simulink model "mpc_model_delayed"  (R2019a)
settings: Solver=FixedStepAuto  StartTime=0.0  StopTime=Tfinal  RelTol=1e-3
values from neighbouring files (symbols this model uses):
  A = [-0.0285 -0.0014; -0.0371 -0.1476]    [model.m]
  DCLINK_Cap = 1000e-12    (= 1e-09)    [mpc_model_parameters.m]    (also in mpc_model_parameters_dual_module.m = 0.001)
  FaultTime = 50    [mpc_model_parameters.m]
  FluxPM = MeanInducedVoltagePeak/(2*pi*100)    [mpc_model_parameters.m]    (also in mpc_model_parameters_dual_module.m)
  Inertia = 1e-2    (= 0.01)    [mpc_model_parameters.m]    (also in mpc_model_parameters_dual_module.m)
  Ls = 3.5e-3    (= 0.0035)    [MPC_id_iq.m]    (also in mpc_model_parameters.m = 0.00351; mpc_model_parameters_dual_module.m = 0.00343)
  PolePairs = 10    [mpc_model_parameters.m]    (also in mpc_model_parameters_dual_module.m)
  Rin = 1e-3    (= 0.001)    [mpc_model_parameters.m]    (also in mpc_model_parameters_dual_module.m)
  Rs = 0.531    [Loss_Distribution.m]    (also in MPC_id_iq.m; mpc_model_parameters.m = 0.321; mpc_model_parameters_dual_module.m = 0.539)
  Sampling_time = 1e-6    (= 1e-06)    [mpc_model_parameters.m]    (also in mpc_model_parameters_dual_module.m)
  SpeedRef1 = 50    [mpc_model_parameters.m]    (also in mpc_model_parameters_dual_module.m = 35)
  SpeedRef2 = 100    [mpc_model_parameters.m]    (also in mpc_model_parameters_dual_module.m = 35)
  SpeedRefUpdateTime = 0.25    [mpc_model_parameters.m]    (also in mpc_model_parameters_dual_module.m = 1.75)
  Tload1 = 5    [mpc_model_parameters.m]    (also in mpc_model_parameters_dual_module.m = 30)
  Tload2 = 10    [mpc_model_parameters.m]    (also in mpc_model_parameters_dual_module.m = 63.6619772368)
  TloadUpdateTime = 0.5    [mpc_model_parameters.m]    (also in mpc_model_parameters_dual_module.m)
  Vdc = 50    [mpc_model_parameters.m]    (also in mpc_model_parameters_dual_module.m = 40)
  Vin = Vdc + Rin*(Pout/Vdc)    (= 50.04)    [mpc_model_parameters.m]    (also in mpc_model_parameters_dual_module.m = 40.05)
  ViscousFriction = 1e-3    (= 0.001)    [mpc_model_parameters.m]    (also in mpc_model_parameters_dual_module.m)
undefined symbols (not defined in the file or in its folder): DiscIntNeverNeededParam
libraries: powerlib x16, dspsigops x16, dspswit3 x10, powerlib_meascontrol x3, dspstat3 x3, simulink x2
settings Model: Creator=hakan  LastModifiedBy=hakan
settings SolverCC: ZeroCrossAlgorithm=Adaptive
settings DebuggingCC: IgnoredZcDiagnostic=none

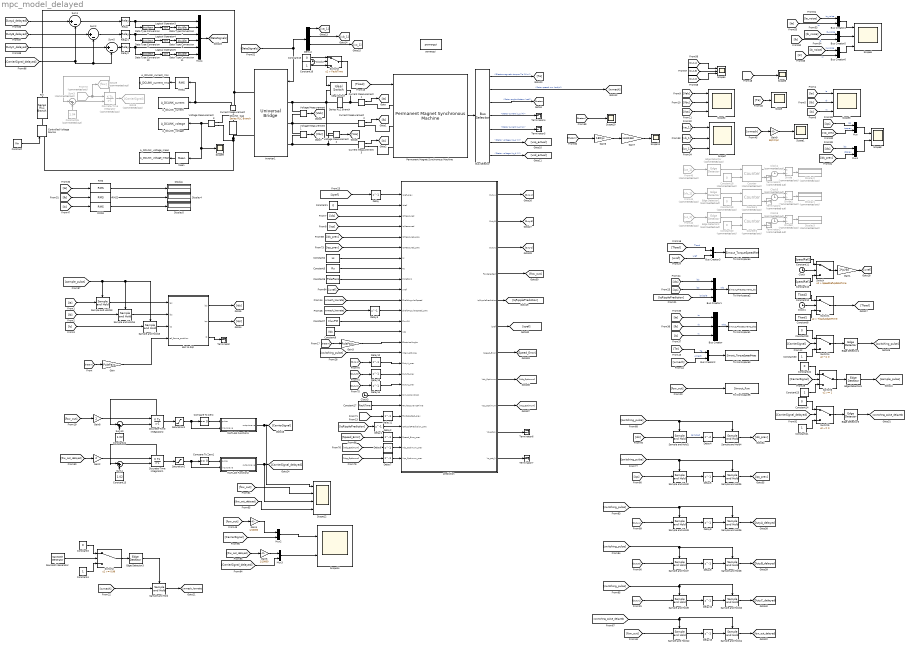
== system mpc_model_delayed ==
  A_DCLINK_current : ToWorkspace  VariableName=A_DCLINK_current  SaveFormat=Structure With Time  SampleTime=-1
  A_DCLINK_current_rms : ToWorkspace  VariableName=A_DCLINK_current_rms  SaveFormat=Structure With Time  SampleTime=-1
  A_DCLINK_voltage : ToWorkspace  VariableName=A_DCLINK_voltage  SaveFormat=Structure With Time  SampleTime=-1
  A_DCLINK_voltage_mean : ToWorkspace  VariableName=A_DCLINK_voltage_mean  SaveFormat=Structure With Time  SampleTime=-1
  Bus Creator : BusCreator  Inputs=3
  Bus Creator1 : BusCreator  Inputs=3
  Bus Creator{2..6} (5 alike) : BusCreator  Inputs=2
  Bus Selector : BusSelector  OutputSignals=Electromagnetic torque Te (N*m),Rotor speed wm (rad/s),Rotor angle thetam (rad),Stator current is_q (A),Stator current is_d (A),Stator voltage Vs_q (V),Stator voltage Vs_d (V)
  Clock{,1..3} (4 alike) : Clock
  Clock4 : Clock  Commented=on
  Clock5 : Clock  Commented=on
  Clock6 : Clock  Commented=on
  Compare To Zero : simulink/Logic and Bit Operations/Compare To Zero  relop===  OutDataTypeStr=boolean
  Compare To Zero1 : simulink/Logic and Bit Operations/Compare To Zero  relop===  OutDataTypeStr=boolean
  Constant : Constant  Value=Vin
  Constant{1,3,14..15,22,29} (6 alike) : Constant  Value=0
  Constant10 : Constant  Value=SpeedRef1
  Constant11 : Constant  Value=SpeedRef2
  Constant12 : Constant  Value=Tload2
  Constant13 : Constant  Value=1.02
  Constant{4,16,21,23,30} (5 alike) : Constant
  Constant17 : Constant  Value=FaultTime
  Constant18 : Constant  Commented=on  Value=0
  Constant19 : Constant  Commented=on  Value=0
  Constant2 : Constant  Value=Ls
  Constant20 : Constant  Commented=on  Value=0
  Constant24 : Constant  Value=1.02
  Constant26 : Constant  Commented=on  Value=1.04
  Constant5 : Constant  Value=Rs
  Constant6 : Constant  Value=PolePairs
  Constant7 : Constant  Value=FluxPM
  Constant8 : Constant  Value=Tload1
  Constant9 : Constant  Value=Vdc
  Controlled Voltage Source : powerlib/Electrical Sources/Controlled Voltage Source  Initialize=on  Source_Type=DC  Amplitude=Vin  Phase=0  Frequency=0  Measurements=None
      settings: SourceProductName=Simscape Electrical
  Counter : dspswit3/Counter  Commented=on  Direction=Up  CountEvent=Rising edge  CounterSize=User defined  MaxCount=9999999999999999999  InitialCount=0  Output=Count and Hit  HitValue=32  ResetInput=on  SamplesPerFrame=1  Ts=1  CntDtype=double  HitDtype=Logical
  Counter1 : dspswit3/Counter  Commented=on  Direction=Up  CountEvent=Rising edge  CounterSize=User defined  MaxCount=9999999999999999999  InitialCount=0  Output=Count and Hit  HitValue=32  ResetInput=on  SamplesPerFrame=1  Ts=1  CntDtype=double  HitDtype=Logical
  Counter2 : dspswit3/Counter  Commented=on  Direction=Up  CountEvent=Rising edge  CounterSize=User defined  MaxCount=9999999999999999999  InitialCount=0  Output=Count and Hit  HitValue=32  ResetInput=on  SamplesPerFrame=1  Ts=1  CntDtype=double  HitDtype=Logical
  Current Measurement{,1..3} (4 alike) : powerlib/Measurements/Current Measurement  PhasorSimulation=off  OutputType=Complex  PSBequivalent=0
      settings: SourceProductName=Simscape Electrical
  DCLINK_Cap : powerlib/Elements/Series RLC Branch  LConnTagsString=__new0  RConnTagsString=__new0  BranchType=C  Resistance=1  Inductance=1e-3  SetiL0=off  InitialCurrent=0  Capacitance=DCLINK_Cap  Setx0=on  InitialVoltage=Vin  Measurements=None
      settings: SourceProductName=Simscape Electrical
  Data Type Conversion10 : DataTypeConversion  OutDataTypeStr=boolean
  Data Type Conversion11 : DataTypeConversion  OutDataTypeStr=double
  Data Type Conversion6 : DataTypeConversion  OutDataTypeStr=boolean
  Data Type Conversion7 : DataTypeConversion  OutDataTypeStr=double
  Data Type Conversion8 : DataTypeConversion  OutDataTypeStr=boolean
  Data Type Conversion9 : DataTypeConversion  OutDataTypeStr=double
  Delay{,1..3,5..15} (15 alike) : Delay  DelayLength=1
  Delay4 : Delay
  Demux : Demux  Outputs=6
  Discrete-Time Integrator : DiscreteIntegrator  Commented=on  ExternalReset=falling  SampleTime=-1  ShowStatePort=on  ICPrevOutput=DiscIntNeverNeededParam  ICPrevScaledInput=DiscIntNeverNeededParam
  Discrete-Time Integrator1 : DiscreteIntegrator  ExternalReset=falling  SampleTime=Sampling_time  UpperSaturationLimit=1  LowerSaturationLimit=0  ShowStatePort=on  ICPrevOutput=DiscIntNeverNeededParam  ICPrevScaledInput=DiscIntNeverNeededParam
  Discrete-Time Integrator2 : DiscreteIntegrator  ExternalReset=falling  SampleTime=Sampling_time  UpperSaturationLimit=1  LowerSaturationLimit=0  ShowStatePort=on  ICPrevOutput=DiscIntNeverNeededParam  ICPrevScaledInput=DiscIntNeverNeededParam
  Display : Display
  Display1 : Display  Commented=on
  Display2 : Display  Commented=on
  Display3 : Display  Commented=on
  Display4 : Display
  Display5 : Display
  Divide : Product  Commented=on  Inputs=*/
  Divide1 : Product  Commented=on  Inputs=*/
  Divide2 : Product  Commented=on  Inputs=*/
  Edge Detector : dspswit3/Edge Detector  Commented=on  InputProcessing=Columns as channels (frame based)
      settings: SourceProductName=DSP System Toolbox  SourceProductBaseCode=DS
  Edge Detector1 : dspswit3/Edge Detector  Commented=on  InputProcessing=Columns as channels (frame based)
      settings: SourceProductName=DSP System Toolbox  SourceProductBaseCode=DS
  Edge Detector2 : dspswit3/Edge Detector  Commented=on  InputProcessing=Columns as channels (frame based)
      settings: SourceProductName=DSP System Toolbox  SourceProductBaseCode=DS
  Edge Detector{3..6} (4 alike) : dspswit3/Edge Detector  InputProcessing=Columns as channels (frame based)
      settings: SourceProductName=DSP System Toolbox  SourceProductBaseCode=DS
  From40 : From  Commented=on  GotoTag=va_1
  From41 : From  Commented=on  GotoTag=vb_1
  From42 : From  Commented=on  GotoTag=vc_1
  From72 : From  Commented=on  GotoTag=fsw_out
  Gain : Gain  Gain=PolePairs
  Gain1 : Gain  Gain=2*pi/60
  Gain2 : Gain  Gain=2
  Gain3 : Gain  Gain=PolePairs
  Gain4 : Gain  Gain=1/10000
  Gain5 : Gain  Gain=1/10000
  Gain6 : Gain  Gain=180/pi
  Gain7 : Gain  Gain=14400/360
  Gain8 : Gain  Gain=2
  Gain9 : Gain  Gain=60/(2*pi)
  Goto29 : Goto  Commented=on  GotoTag=fsw
  Goto9 : Goto  Commented=on  GotoTag=CarrierSignal
  Ideal Switch : powerlib/Power Electronics/Ideal Switch  Ron=0.001  Lon=0  IC=0  Rs=1e5  Cs=inf  Measurements=on
      settings: SourceProductName=Simscape Electrical
  Inverter1 : powerlib/Power Electronics/Universal Bridge  Arms=3  SnubberResistance=1e5  SnubberCapacitance=inf  Device=IGBT / Diodes  Ron=0.65e-3  Lon=0  ForwardVoltages="[  0  0  ]"  ForwardVoltage=0  GTOparameters=[ 10e-6 , 20e-6 ]  IGBTparameters=[ 1e-6 , 2e-6 ]  Measurements=All voltages and currents  Measurements_2=None  converterType=Rectifier
      settings: SourceProductName=Simscape Electrical
  Logical Operator3 : Logic  Operator=NOT  AllPortsSameDT=off  OutDataTypeStr=boolean
  Logical Operator4 : Logic  Operator=NOT  AllPortsSameDT=off  OutDataTypeStr=boolean
  Logical Operator5 : Logic  Operator=NOT  AllPortsSameDT=off  OutDataTypeStr=boolean
  MATLAB Function1 : MATLAB Function  TreatAsAtomicUnit=on
  MATLAB Function2 : MATLAB Function  TreatAsAtomicUnit=on
  Mean : powerlib_meascontrol/Measurements/Mean  Freq=THD_mean_frequency  Vinit=0  Ts=0
      settings: SourceProductName=Simscape Electrical
  Mux{,1..3} (4 alike) : Mux  Inputs=2
  Mux4 : Mux  Inputs=6
  Permanent Magnet Synchronous Machine : powerlib/Machines/Permanent Magnet Synchronous Machine  NbPhases=3  FluxDistribution=Sinusoidal  RotorType=Round  MechanicalLoad=Torque Tm  PresetModel=No  ShowDetailedParameters=on  MeasurementBus=off  Resistance=Rs  Inductance=8.5e-3  dqInductances=[3.1e-3,3.6e-3]  La=Ls_Machine  MachineConstant=Voltage Constant (V_peak L-L / krpm)  Flux=0.18074  VoltageCst=VoltageConstant  TorqueCst=2.7111  Flat=120  Mechanical=[Inertia ViscousFriction PolePairs 0]  PolePairs=4  InitialConditions=[0*100*2*pi/60,0, 0,0]  InitialConditions5ph=[0 0 0 0 0 0]  TsPowergui=0  TsBlock=-1  RefAngle=90 degrees behind phase A axis (modified Park)
  RMS : dspstat3/RMS  run=off  directionMode=Each column  dimension=1  InputProcessing=Columns as channels (frame based)  reset_popup=None
  RMS1 : powerlib_meascontrol/Measurements/RMS  TrueRMS=on  Freq=Load_Nominal_Freq  RMSInit=10  Ts=0
      settings: SourceProductName=Simscape Electrical
  RMS2 : dspstat3/RMS  run=off  directionMode=Each column  dimension=1  InputProcessing=Columns as channels (frame based)  reset_popup=None
  RMS3 : dspstat3/RMS  run=off  directionMode=Each column  dimension=1  InputProcessing=Columns as channels (frame based)  reset_popup=None
  Relay : Relay
  Relay1 : Relay
  Relay2 : Relay
  Rin : powerlib/Elements/Series RLC Branch  LConnTagsString=__new0  RConnTagsString=__new0  BranchType=R  Resistance=Rin  Inductance=1e-3  SetiL0=off  InitialCurrent=0  Capacitance=1000e-6  Setx0=off  InitialVoltage=0  Measurements=None
      settings: SourceProductName=Simscape Electrical
  Sample and Hold{,1..15} (16 alike) : dspsigops/Sample and Hold  trig=Rising edge  initCond=0  latchinput=off
  Saturation1 : Saturate  UpperLimit=1  LowerLimit=0
  Saturation2 : Saturate  UpperLimit=1  LowerLimit=0
  Sawtooth Generator : powerlib_meascontrol/Pulse & Signal Generators/Sawtooth Generator  Freq=100  Phase=180  Ts=0
      settings: SourceProductName=Simscape Electrical
  Scope{,1,5,9..11} (6 alike) : Scope
  Scope12 : Scope  NumInputPorts=4
  Scope14 : Scope  NumInputPorts=2
  Scope{2..4,6..7} (5 alike) : Scope  NumInputPorts=3
  Scope8 : Scope  NumInputPorts=2
  Series RLC Branch : powerlib/Elements/Series RLC Branch  LConnTagsString=__new0  RConnTagsString=__new0  BranchType=R  Resistance=5000  Inductance=1e-3  SetiL0=off  InitialCurrent=0  Capacitance=1e-6  Setx0=off  InitialVoltage=0  Measurements=None
      settings: SourceProductName=Simscape Electrical
  Sum1 : Sum  Inputs=|+-
  Sum10 : Sum  Inputs=|-+
  Sum2 : Sum  Inputs=|+-
  Sum3 : Sum  Commented=on  Inputs=|-+
  Sum4 : Sum  Inputs=|-+
  Sum5 : Sum  Inputs=|+-
  Switch : Switch  Criteria=u2 > Threshold  Threshold=SpeedRefUpdateTime
  Switch1 : Switch  Criteria=u2 > Threshold  Threshold=TloadUpdateTime
  Switch2 : Switch  Threshold=0.99
  Switch3 : Switch  Criteria=u2 > Threshold  Threshold=FaultTime
  Switch4 : Switch  Criteria=u2 ~= 0
  Switch5 : Switch  Criteria=u2 ~= 0
  Switch6 : Switch  Threshold=1
  Terminator{,4..7} (5 alike) : Terminator
  Terminator1 : Terminator  Commented=on
  Terminator2 : Terminator  Commented=on
  Terminator3 : Terminator  Commented=on
  To Workspace1 : ToWorkspace  VariableName=Simout_PhaseCurrents_abc  SaveFormat=Timeseries  SampleTime=-1
  To Workspace2 : ToWorkspace  VariableName=Simout_PhaseCurrents_dq  SaveFormat=Timeseries  SampleTime=-1
  To Workspace3 : ToWorkspace  VariableName=Simout_TorqueSpeedMeas  SaveFormat=Timeseries  SampleTime=-1
  To Workspace4 : ToWorkspace  VariableName=Simout_TorqueSpeedRef  SaveFormat=Timeseries  SampleTime=-1
  To Workspace5 : ToWorkspace  VariableName=Simout_Fsw  SaveFormat=Timeseries  SampleTime=-1
  Voltage Measurement{,1..3} (4 alike) : powerlib/Measurements/Voltage Measurement  PhasorSimulation=off  OutputType=Complex  PSBequivalent=0
      settings: SourceProductName=Simscape Electrical
  abc to dq0 : MATLAB Function  TreatAsAtomicUnit=on
  powergui : powerlib/powergui  Priority=1  SimulationMode=Discrete  SampleTime=Sampling_time  frequency=60  Iterations=50  frequencyindice=0  Pbase=100e6  ErrMax=1e-4  UnitsV=kV  UnitsW=MW  buscounter=0  FunctionMessages=off  echomessages=off  EnableUseOfTLC=off  CurrentSourceSwitches=off  DisableSnubberDevices=off  DisableRonSwitches=off  DisableVfSwitches=off  DisplayEquations=off  AutomaticDiscreteSolvers=off  SolverType=Tustin/Backward Euler (TBE)  Interpol=off  ExternalGateDelay=off  methode=off  Ts=100  x0status=blocks  SPID=on  SwTol=0  HookPort=off  NonlinearTolerance=0  nMaxIteration=15  ContinueOnMaxIteration=off  RestoreLinks=warning  ResistiveCurrentMeasurement=off  Frange=[0:2:500]  Ylog=off  Xlog=on  ShowGrid=off  save=off  variable=ZData  structure=0  ZoomFFT=off  StartTime=0.0  cycles=1  DisplayStyle=1  fundamental=60  FreqAxis=off  MaxFrequency=1000  frequencyindicesteady=1  RmsSteady=1  display=off
      settings: SourceProductName=Simscape Electrical
  prediction : MATLAB Function  TreatAsAtomicUnit=on
  wires:
  Voltage Measurement3/1 -> Scope9/1, Mean/1, A_DCLINK_voltage/1
  RMS1/1 -> A_DCLINK_current_rms/1
  Constant/1 -> Controlled Voltage Source/1
  Mean/1 -> A_DCLINK_voltage_mean/1
  Current Measurement/1 -> RMS1/1, A_DCLINK_current/1
  Permanent Magnet Synchronous Machine/1 -> Bus Selector/1
  Bus Selector/1 -> [Te]  "<Electromagnetic torque Te (N*m)>"
  Bus Selector/2 -> [wmech]  "<Rotor speed wm (rad/s)>"
  Current Measurement1/1 -> [Ia]
  Current Measurement2/1 -> [Ib]
  Current Measurement3/1 -> [Ic]
  Bus Selector/3 -> [thetam]  "<Rotor angle thetam (rad)>"
  Bus Selector/4 -> Terminator4/1  "<Stator current is_q (A)>"
  Bus Selector/5 -> Terminator5/1  "<Stator current is_d (A)>"
  [ids] -> prediction/3(IdMeasured)
  [iqs] -> prediction/4(IqMeasured)
  Constant2/1 -> prediction/7(Ls)
  Voltage Measurement/1 -> [Vab]
  Voltage Measurement1/1 -> [Vbc]
  Voltage Measurement2/1 -> [Vca]
  Bus Selector/6 -> [vsq_actual]  "<Stator voltage Vs_q (V)>"
  Bus Selector/7 -> [vsd_actual]  "<Stator voltage Vs_d (V)>"
  [Vca] -> Scope2/3
  [Vbc] -> Scope2/2
  [Vab] -> Scope2/1
  Constant5/1 -> prediction/8(Rs)
  Constant6/1 -> prediction/9(PolePairs)
  [wmech_lowrate] -> prediction/11(ShaftAngularSpeed)
  Constant7/1 -> prediction/13(FluxPM)
  Constant9/1 -> prediction/14(Vdc)
  Gain3/1 -> prediction/15(ElectricalAngle)
  [thetam] -> Gain3/1
  [Tload] -> Permanent Magnet Synchronous Machine/1
  [iqs] -> Bus Creator1/2  "iqs"
  [ids] -> Bus Creator1/1  "ids"
  Constant10/1 -> Switch/3
  Constant11/1 -> Switch/1
  Switch/1 -> Gain1/1
  Clock/1 -> Switch/2
  Clock1/1 -> Switch1/2
  Constant12/1 -> Switch1/1
  Constant8/1 -> Switch1/3
  Switch1/1 -> [Tload]
  Bus Creator/1 -> To Workspace1/1  "Iabc"
  Bus Creator1/1 -> To Workspace2/1  "Idq"
  Bus Creator2/1 -> To Workspace3/1
  Gain1/1 -> [wref]
  [Tload] -> Bus Creator3/1  "Tload"
  [wref] -> Bus Creator3/2  "wref"
  Bus Creator3/1 -> To Workspace4/1
  [switching_pulse] -> prediction/16(InterruptPulse)
  Clock2/1 -> Switch3/2
  Constant15/1 -> Switch3/1
  Constant16/1 -> Switch3/3
  Switch3/1 -> Ideal Switch/1
  Clock3/1 -> prediction/20(SimulationClock)
  Constant17/1 -> prediction/21(FaultOccuranceTime)
  [va_1] -> Scope7/1
  [vb_1] -> Scope7/2
  [vc_1] -> Scope7/3
  Edge Detector/1 -> Counter/1
  Constant18/1 -> Counter/2
  Counter/1 -> Divide/1
  Clock4/1 -> Divide/2
  Divide/1 -> Display2/1
  [Ib] -> Bus Creator/2  "Ib"
  [Ia] -> Bus Creator/1  "Ia"
  [Ic] -> Bus Creator/3  "Ic"
  [Ib] -> Scope3/2  "Ib"
  [Ic] -> Scope3/3  "Ic"
  [Ia] -> Scope3/1  "Ia"
  Counter/2 -> Terminator1/1
  From40/1 -> Edge Detector/1
  From41/1 -> Edge Detector1/1
  Counter1/2 -> Terminator2/1
  Divide1/1 -> Display1/1
  Clock5/1 -> Divide1/2
  Counter1/1 -> Divide1/1
  Constant19/1 -> Counter1/2
  Edge Detector1/1 -> Counter1/1
  Edge Detector2/1 -> Counter2/1
  Constant20/1 -> Counter2/2
  Counter2/1 -> Divide2/1
  Clock6/1 -> Divide2/2
  Divide2/1 -> Display3/1
  Counter2/2 -> Terminator3/1
  From42/1 -> Edge Detector2/1
  [Te] -> Bus Creator2/1  "Te"
  [wmech] -> Bus Creator2/2  "wmech"
  [Te] -> Scope/1
  [wmech] -> Gain9/1
  prediction/1(DutyA) -> [DutyA]
  prediction/3(DutyC) -> [DutyC]
  prediction/2(DutyB) -> [DutyB]
  [DutyB] -> Scope4/2
  [DutyA] -> Scope4/1
  [DutyC] -> Scope4/3
  Constant26/1 -> Sum3/2
  From72/1 -> Goto29/1, Discrete-Time Integrator/1
  Discrete-Time Integrator/State -> Sum3/1
  Sum3/1 -> Discrete-Time Integrator/2
  Switch4/1 -> Edge Detector4/1
  Constant30/1 -> Switch4/3
  Constant29/1 -> Switch4/1
  [GateSignals] -> Inverter1/1, Demux/1
  Demux/1 -> [va_1]
  Demux/3 -> [vb_1]
  prediction/4(FswSelected) -> [fsw_out]
  Delay11/1 -> prediction/22(FswSelected_prev)
  [fsw_out] -> Delay11/1
  [DutyB] -> Delay13/1
  [DutyA] -> Delay12/1
  [DutyC] -> Delay14/1
  Delay13/1 -> prediction/18(DutyB_prev)
  Delay12/1 -> prediction/17(DutyA_prev)
  Delay14/1 -> prediction/19(DutyC_prev)
  Discrete-Time Integrator/1 -> Goto9/1
  [CarrierSignal] -> Switch4/2
  Demux/5 -> [vc_1]
  [IqRipplePrediction] -> Delay1/1
  Delay1/1 -> prediction/23(IqRipplePrediction_prev)
  [CarrierSignal_delayed] -> Sum2/2, Sum5/2, Sum1/2
  Logical Operator4/1 -> Data Type Conversion9/1
  [DutyA_delayed] -> Sum1/1
  Data Type Conversion8/1 -> Logical Operator4/1
  Data Type Conversion10/1 -> Logical Operator5/1
  Relay1/1 -> Data Type Conversion8/1, Mux4/3
  Relay2/1 -> Data Type Conversion10/1, Mux4/5
  Data Type Conversion6/1 -> Logical Operator3/1
  Sum1/1 -> Relay/1
  Data Type Conversion11/1 -> Mux4/6
  [DutyC_delayed] -> Sum5/1
  Relay/1 -> Mux4/1, Data Type Conversion6/1
  Data Type Conversion9/1 -> Mux4/4
  Sum5/1 -> Relay2/1
  Logical Operator3/1 -> Data Type Conversion7/1
  Logical Operator5/1 -> Data Type Conversion11/1
  Sum2/1 -> Relay1/1
  Mux4/1 -> [GateSignals]
  [DutyB_delayed] -> Sum2/1
  Data Type Conversion7/1 -> Mux4/2
  [fsw_out] -> Scope5/1
  Discrete-Time Integrator2/State -> Sum10/1
  Gain8/1 -> Discrete-Time Integrator2/1
  Sum10/1 -> Discrete-Time Integrator2/2
  [fsw_out] -> Gain8/1
  Saturation1/1 -> MATLAB Function1/2(inputwave), Compare To Zero/1
  Constant24/1 -> Sum10/2
  Discrete-Time Integrator2/1 -> Saturation1/1
  Compare To Zero/1 -> MATLAB Function1/1(pulse)
  MATLAB Function1/1(outputwave) -> Scope12/1, [CarrierSignal]
  [fsw_out] -> To Workspace5/1
  [IqRipplePrediction] -> Bus Creator1/3  "iqripple"
  Constant1/1 -> prediction/2(idref)
  prediction/5(IqRipplePrediction) -> [IqRipplePrediction]
  Switch2/1 -> Edge Detector3/1
  Edge Detector3/1 -> Sample and Hold/Trigger
  Constant4/1 -> Switch2/3
  Sawtooth Generator/1 -> Switch2/2
  Constant3/1 -> Switch2/1
  [wmech] -> Sample and Hold/1
  Sample and Hold/1 -> [wmech_lowrate]
  [Ia] -> RMS/1
  [Ib] -> RMS2/1
  [Ic] -> RMS3/1
  RMS/1 -> Display/1
  RMS2/1 -> Display4/1
  RMS3/1 -> Display5/1
  abc to dq0/2(iqs) -> [iqs]
  Gain/1 -> abc to dq0/4(ref_frame_position)
  abc to dq0/1(ids) -> [ids]
  abc to dq0/3(i0) -> Terminator/1
  [thetam] -> Gain/1
  [Ia_noise] -> Bus Creator4/1  "Ia_noise"
  [Ia] -> Bus Creator4/2  "Ia"
  [Ib] -> Bus Creator5/2  "Ib"
  [Ib_noise] -> Bus Creator5/1  "Ib_noise"
  [Ic_noise] -> Bus Creator6/1  "Ic_noise"
  [Ic] -> Bus Creator6/2  "Ic"
  Bus Creator5/1 -> Scope6/2
  Bus Creator4/1 -> Scope6/1
  Bus Creator6/1 -> Scope6/3
  prediction/6(iqref) -> [iqref]
  Delay/1 -> prediction/1(iqref_prev)
  [iqref] -> Delay/1
  [wref] -> prediction/10(wref)
  [wmech_lowrate] -> Delay3/1
  prediction/7(Speed_Error) -> [Speed_Error]
  Delay2/1 -> prediction/24(Speed_Error_prev)
  [Speed_Error] -> Delay2/1
  Delay3/1 -> prediction/12(ShaftAngularSpeed_prev)
  [thetam] -> Scope10/1
  [thetam] -> Gain6/1
  Gain6/1 -> Gain7/1
  Gain7/1 -> Scope11/1
  Edge Detector4/1 -> [switching_pulse]
  [switching_pulse] -> Sample and Hold4/Trigger, Sample and Hold1/Trigger
  [ids] -> Sample and Hold1/1
  [iqs] -> Sample and Hold2/1
  [switching_pulse] -> Sample and Hold5/Trigger, Sample and Hold2/Trigger
  Sample and Hold1/1 -> Delay4/1  "sampled"
  Sample and Hold2/1 -> Delay5/1
  Delay5/1 -> Sample and Hold5/1
  Delay4/1 -> Sample and Hold4/1
  Sample and Hold4/1 -> [ids_prev]
  Sample and Hold5/1 -> [iqs_prev]
  [ids_prev] -> prediction/5(IdMeasured_prev)
  [iqs_prev] -> prediction/6(IqMeasured_prev)
  prediction/8(Vds_Optimum) -> [Vds_Optimum]
  prediction/9(Vqs_Optimum) -> [Vqs_Optimum]
  [Vds_Optimum] -> Delay6/1
  [Vqs_Optimum] -> Delay7/1
  Delay6/1 -> prediction/25(Vds_Optimum_prev)
  Delay7/1 -> prediction/26(Vqs_Optimum_prev)
  prediction/10(Vd_est_1) -> Terminator6/1
  prediction/11(Vq_est_1) -> Terminator7/1
  Gain9/1 -> Scope1/1
  [iqs] -> Mux/1  "iqs"
  [iqs_prev] -> Mux/2  "iqsprev"
  Mux/1 -> Scope8/1
  Mux1/1 -> Scope8/2
  [ids] -> Mux1/1  "ids"
  [ids_prev] -> Mux1/2  "idsprev"
  Sample and Hold6/1 -> [DutyA_delayed]
  Delay8/1 -> Sample and Hold6/1
  Sample and Hold3/1 -> Delay8/1
  [switching_pulse] -> Sample and Hold6/Trigger, Sample and Hold3/Trigger
  [DutyA] -> Sample and Hold3/1
  [DutyB] -> Sample and Hold7/1
  [switching_pulse] -> Sample and Hold7/Trigger, Sample and Hold8/Trigger
  Sample and Hold7/1 -> Delay9/1
  Delay9/1 -> Sample and Hold8/1
  Sample and Hold8/1 -> [DutyB_delayed]
  Sample and Hold10/1 -> [DutyC_delayed]
  Delay10/1 -> Sample and Hold10/1
  Sample and Hold9/1 -> Delay10/1
  [switching_pulse] -> Sample and Hold10/Trigger, Sample and Hold9/Trigger
  [DutyC] -> Sample and Hold9/1
  [fsw_out] -> Sample and Hold12/1
  [switching_pulse_delayed] -> Sample and Hold11/Trigger, Sample and Hold12/Trigger
  Sample and Hold11/1 -> [fsw_out_delayed]
  Sample and Hold12/1 -> Delay15/1
  Delay15/1 -> Sample and Hold11/1
  MATLAB Function2/1(outputwave) -> Scope12/3, [CarrierSignal_delayed]
  Compare To Zero1/1 -> MATLAB Function2/1(pulse)
  Discrete-Time Integrator1/1 -> Saturation2/1
  Constant13/1 -> Sum4/2
  Saturation2/1 -> Compare To Zero1/1, MATLAB Function2/2(inputwave)
  [fsw_out_delayed] -> Gain2/1
  Sum4/1 -> Discrete-Time Integrator1/2
  Gain2/1 -> Discrete-Time Integrator1/1
  Discrete-Time Integrator1/State -> Sum4/1
  [fsw_out] -> Scope12/2
  [fsw_out_delayed] -> Scope12/4
  Edge Detector5/1 -> [switching_pulse_delayed]
  [CarrierSignal_delayed] -> Switch5/2
  Constant14/1 -> Switch5/1
  Constant21/1 -> Switch5/3
  Switch5/1 -> Edge Detector5/1
  Mux2/1 -> Scope14/1
  Mux3/1 -> Scope14/2
  [fsw_out_delayed] -> Gain5/1
  [fsw_out] -> Gain4/1
  [CarrierSignal] -> Mux2/2
  [CarrierSignal_delayed] -> Mux3/2
  Gain4/1 -> Mux2/1
  Gain5/1 -> Mux3/1
  Edge Detector6/1 -> [sample_pulse]
  [CarrierSignal] -> Switch6/2
  Constant22/1 -> Switch6/1
  Constant23/1 -> Switch6/3
  Switch6/1 -> Edge Detector6/1
  [Ia] -> Sample and Hold13/1
  Sample and Hold13/1 -> abc to dq0/1(ias)
  Sample and Hold14/1 -> abc to dq0/2(ibs)
  [Ib] -> Sample and Hold14/1
  Sample and Hold15/1 -> abc to dq0/3(ics)
  [Ic] -> Sample and Hold15/1
  [sample_pulse] -> Sample and Hold15/Trigger, Sample and Hold14/Trigger, Sample and Hold13/Trigger
  connections:
  Rin/LConn1 -- Current Measurement/RConn1 -- Inverter1/RConn1
  Controlled Voltage Source/LConn1 -- Voltage Measurement3/LConn2 -- DCLINK_Cap/RConn1 -- Inverter1/RConn2
  DCLINK_Cap/LConn1 -- Current Measurement/LConn1 -- Voltage Measurement3/LConn1
  Controlled Voltage Source/RConn1 -- Rin/RConn1
  Voltage Measurement2/LConn2 -- Ideal Switch/LConn1 -- Series RLC Branch/LConn1 -- Voltage Measurement/LConn1 -- Inverter1/LConn1
  Current Measurement2/LConn1 -- Voltage Measurement1/LConn1 -- Voltage Measurement/LConn2 -- Inverter1/LConn2
  Inverter1/LConn3 -- Voltage Measurement1/LConn2 -- Voltage Measurement2/LConn1 -- Current Measurement3/LConn1
  Current Measurement3/RConn1 -- Permanent Magnet Synchronous Machine/LConn3
  Permanent Magnet Synchronous Machine/LConn2 -- Current Measurement2/RConn1
  Permanent Magnet Synchronous Machine/LConn1 -- Current Measurement1/RConn1
  Current Measurement1/LConn1 -- Ideal Switch/RConn1 -- Series RLC Branch/RConn1

== matlab function mpc_model_delayed/prediction ==
  data: DutyA output; DutyB output; DutyC output; iqref_prev input; idref input; IdMeasured input; IqMeasured input; IdMeasured_prev input; IqMeasured_prev input; Ls input; Rs input; PolePairs input; wref input; ShaftAngularSpeed input; ShaftAngularSpeed_prev input; FluxPM input; Vdc input; ElectricalAngle input; InterruptPulse input; DutyA_prev input; DutyB_prev input; DutyC_prev input; SimulationClock input; FaultOccuranceTime input; FswSelected_prev input; FswSelected output; IqRipplePrediction output; IqRipplePrediction_prev input; iqref output; Speed_Error_prev input; Speed_Error output; Vds_Optimum output; Vqs_Optimum output; Vds_Optimum_prev input; Vqs_Optimum_prev input; Vd_est_1 output; Vq_est_1 output
function [DutyA, DutyB, DutyC, FswSelected, IqRipplePrediction,iqref,Speed_Error,Vds_Optimum,Vqs_Optimum,Vd_est_1,Vq_est_1] = fcn(iqref_prev,idref,IdMeasured, IqMeasured, IdMeasured_prev, IqMeasured_prev, Ls, Rs,PolePairs,wref, ShaftAngularSpeed,ShaftAngularSpeed_prev, FluxPM,Vdc,ElectricalAngle,InterruptPulse,DutyA_prev, DutyB_prev, DutyC_prev, SimulationClock,FaultOccuranceTime,FswSelected_prev, IqRipplePrediction_prev,Speed_Error_prev,Vds_Optimum_prev,Vqs_Optimum_prev)
Ld = Ls;
Lq = Ls;
Iq_Rated = 11.7362; %this is the rated value of the IqMeasured
% cost = zeros(1,8);
% VdPrediction_1 = zeros(1,8);
% VqPrediction_1 = zeros(1,8);
% FswOptions = [5000; 10000; 15000; 20000; 25000; 30000; 35000; 40000];
FswMax = 10000;
FswOptions = 1000:1000:FswMax;
cost = zeros(1,numel(FswOptions));
% VdPrediction_1 = zeros(1,numel(FswOptions));
% VqPrediction_1 = zeros(1,numel(FswOptions));
Vd_est_1 = zeros(1,numel(FswOptions));
Vq_est_1 = zeros(1,numel(FswOptions));
% Vd_est_2 = zeros(1,numel(FswOptions));
% Vq_est_2 = zeros(1,numel(FswOptions));
VdPrediction_2 = zeros(1,numel(FswOptions));
VqPrediction_2 = zeros(1,numel(FswOptions));
IqRipplePredictionArray_1 = zeros(1,numel(FswOptions));
IqRipplePredictionArray_2 = zeros(1,numel(FswOptions));
VoltageDuring_T1_1 = zeros(1,numel(FswOptions));
VoltageDuring_T2_1 = zeros(1,numel(FswOptions));
VoltageDuring_T0_1 = zeros(1,numel(FswOptions));
VoltageDuring_T1_2 = zeros(1,numel(FswOptions));
VoltageDuring_T2_2 = zeros(1,numel(FswOptions));
VoltageDuring_T0_2 = zeros(1,numel(FswOptions));
MagnitudePrediction_1 = zeros(1,numel(FswOptions));
MagnitudePrediction_2 = zeros(1,numel(FswOptions));

SvpwmT1Prediction_1 =  zeros(1,numel(FswOptions));
SvpwmT2Prediction_1 =  zeros(1,numel(FswOptions));
SvpwmT0Prediction_1 =  zeros(1,numel(FswOptions));

SvpwmT1Prediction_2 =  zeros(1,numel(FswOptions));
SvpwmT2Prediction_2 =  zeros(1,numel(FswOptions));
SvpwmT0Prediction_2 =  zeros(1,numel(FswOptions));

ValfaPrediction_1 = zeros(1,numel(FswOptions)); 
VbetaPrediction_1 = zeros(1,numel(FswOptions)); 
ValfaPrediction_2 = zeros(1,numel(FswOptions)); 
VbetaPrediction_2 = zeros(1,numel(FswOptions)); 
maPrediction_1 = zeros(1,numel(FswOptions)); 
maPrediction_2 = zeros(1,numel(FswOptions));

IqDelta_Prediction_During_T1_1 =  zeros(1,numel(FswOptions));
IqDelta_Prediction_During_T2_1 =  zeros(1,numel(FswOptions));
IqDelta_Prediction_During_T0_1 =  zeros(1,numel(FswOptions));
IqDelta_Prediction_During_T1_2 =  zeros(1,numel(FswOptions));
IqDelta_Prediction_During_T2_2 =  zeros(1,numel(FswOptions));
IqDelta_Prediction_During_T0_2 =  zeros(1,numel(FswOptions));
VoltageVectorAnglePredictionMod_1 = zeros(1,numel(FswOptions));
VoltageVectorAnglePrediction_1 = zeros(1,numel(FswOptions));
VoltageVectorAnglePredictionMod_2 = zeros(1,numel(FswOptions));
VoltageVectorAnglePrediction_2 = zeros(1,numel(FswOptions));

IdPrediction_1_array = zeros(1,numel(FswOptions));
IqPrediction_1_array = zeros(1,numel(FswOptions));
IdPrediction_2_array = zeros(1,numel(FswOptions));
IqPrediction_2_array = zeros(1,numel(FswOptions));

Vd_Vq_Kp = 10;
Vd_Vq_Ki = 1;

MinimumCostValue = 1e20;
MinimumCostIndex = -1;

IqRippleCoeff = 100000;
IqRefCoeff = 10000;
IdRefCoeff = 15;
FswCoeff = 1250;
Iq_1_Method1 = 0;
Id_1_Method1 = 0;
Iq_2_Method1 = 0;
Id_2_Method1 = 0;
Kp = 0.35;
Ki = 50;
Ts_PI = 1/40000;
OptimizeForFsws = 0;
if(FswSelected_prev<=0)
    FswSelected_prev = 1000;
end
if(FswSelected_prev==1000)
    OptimizeForFsws = 1:1:2;
else if(FswSelected_prev==10000)
     OptimizeForFsws = 9:1:10;
    else
        OptimizeForFsws = (FswSelected_prev/1000-1):1:(FswSelected_prev/1000+1);
    end
end
% y = y_prev + Kp*(u-u_prev)+Ts/2*Ki*(u+u_prev);
if(InterruptPulse==1)
    Speed_Error =  wref-ShaftAngularSpeed;
    
    iqref = iqref_prev + Kp*(Speed_Error-Speed_Error_prev)+Ts_PI/2*Ki*((Speed_Error+Speed_Error_prev));
%     if(iqref>(2*Iq_Rated))
%         iqref = 2*Iq_Rated;
%     end
%     if(iqref<(-2*Iq_Rated))
%         iqref = -2*Iq_Rated;
%     end
    if(abs(iqref)>(2*Iq_Rated))
        if(iqref>0)
            iqref = (2*Iq_Rated);
        else
            iqref = -(2*Iq_Rated);
        end
    end
%     for i = 1:numel(FswOptions)
    for i = OptimizeForFsws(1):OptimizeForFsws(end)
        %% first prediction      
        
% % %         Vd_est_1(i) = Rs*IdMeasured+Ls*FswOptions(i)*(idref-IdMeasured)-PolePairs*ShaftAngularSpeed*Ls*IqMeasured;
% % %         Vq_est_1(i) = Rs*IqMeasured+Ls*FswOptions(i)*(iqref-IqMeasured)+PolePairs*ShaftAngularSpeed*(Ld*IdMeasured+FluxPM);

        
        
%         MagnitudePrediction_1(i) = sqrt(VdPrediction_1(i)^2+VqPrediction_1(i)^2);
%         
%         ValfaPrediction_1(i) = sin(ElectricalAngle)*VdPrediction_1(i)+cos(ElectricalAngle)*VqPrediction_1(i);
%         VbetaPrediction_1(i) =-cos(ElectricalAngle)*VdPrediction_1(i)+sin(ElectricalAngle)*VqPrediction_1(i);     
%         
%         VoltageVectorAnglePrediction_1(i) = atan2(VbetaPrediction_1(i),ValfaPrediction_1(i))+4*pi;
%         VoltageVectorAnglePredictionMod_1(i) = mod(VoltageVectorAnglePrediction_1(i),pi/3);
%         
%         maPrediction_1(i) = MagnitudePrediction_1(i)/(Vdc/sqrt(3));
%         
%         SvpwmT1Prediction_1(i) = (1/FswOptions(i))*maPrediction_1(i)*sin(pi/3-VoltageVectorAnglePredictionMod_1(i));
%         SvpwmT2Prediction_1(i) = (1/FswOptions(i))*maPrediction_1(i)*sin(VoltageVectorAnglePredictionMod_1(i));
%         SvpwmT0Prediction_1(i) = (1/FswOptions(i))-SvpwmT1Prediction_1(i)-SvpwmT2Prediction_1(i);        
%         
%         VoltageDuring_T1_1(i) = 2/3*Vdc-MagnitudePrediction_1(i);
%         VoltageDuring_T2_1(i) = 2/3*Vdc-MagnitudePrediction_1(i);
%         VoltageDuring_T0_1(i) = -MagnitudePrediction_1(i);
%         
%         IqDelta_Prediction_During_T1_1(i) = VoltageDuring_T1_1(i)*SvpwmT1Prediction_1(i)/Ls;
%         IqDelta_Prediction_During_T2_1(i) = VoltageDuring_T2_1(i)*SvpwmT2Prediction_1(i)/Ls;
%         IqDelta_Prediction_During_T0_1(i) = -VoltageDuring_T0_1(i)*SvpwmT0Prediction_1(i)/Ls;
%         
%         IqRipplePredictionArray_1(i) = IqDelta_Prediction_During_T1_1(i)+IqDelta_Prediction_During_T2_1(i)+IqDelta_Prediction_During_T0_1(i);
        
        %predict the future output
        
%         IdPrediction_1 = IdMeasured + (1/FswOptions(i))*(Vd_est_1(i)/Ld-Rs/Ld*IdMeasured+Lq/Ld*PolePairs*ShaftAngularSpeed*IqMeasured);
%         IqPrediction_1 = IqMeasured + (1/FswOptions(i))*(Vq_est_1(i)/Lq-Rs/Lq*IqMeasured-Ld/Lq*PolePairs*ShaftAngularSpeed*IdMeasured-FluxPM*PolePairs*ShaftAngularSpeed/Lq);
        IdPrediction_1 = IdMeasured + (1/FswOptions(i))*(Vds_Optimum_prev/Ld-Rs/Ld*IdMeasured+Lq/Ld*PolePairs*ShaftAngularSpeed*IqMeasured);
        IqPrediction_1 = IqMeasured + (1/FswOptions(i))*(Vqs_Optimum_prev/Lq-Rs/Lq*IqMeasured-Ld/Lq*PolePairs*ShaftAngularSpeed*IdMeasured-FluxPM*PolePairs*ShaftAngularSpeed/Lq);
%         TePrediction_1 = 1.5*PolePairs*(FluxPM*IqPrediction_1+0*(Ld-Lq)*IdPrediction_1*IqPrediction_1); % reluctance torque component is multiplied by 0, since it caused unreasonable torque values.
                
        IdPrediction_1_array(i) = IdPrediction_1;
        IqPrediction_1_array(i) = IqPrediction_1;
        
        Vd_Vq_Kp = Ls/(2)*FswOptions(i);
        Vd_Vq_Ki = Rs/Ls;
        
        Vd_est_1(i) = Vd_Vq_Kp * (idref-IdPrediction_1) * ( 1 + Vd_Vq_Ki / FswOptions(i) ) + IdMeasured - PolePairs*ShaftAngularSpeed*Ls*IqPrediction_1;
        Vq_est_1(i) = Vd_Vq_Kp * (iqref-IqPrediction_1) * ( 1 + Vd_Vq_Ki / FswOptions(i) ) + IqMeasured + PolePairs*ShaftAngularSpeed*(Ls*IdPrediction_1 + FluxPM);

%         Vd_est_1(i) = Vds_Optimum_prev + Vd_Vq_Kp*Vd_Vq_Ki/ FswOptions(i)*(idref-IdPrediction_1);
%         Vq_est_1(i) = Vqs_Optimum_prev + Vd_Vq_Kp*Vd_Vq_Ki/ FswOptions(i)*(iqref-IqPrediction_1);

        MagnitudePrediction_1(i) = sqrt(Vd_est_1(i)^2+Vq_est_1(i)^2);
        
        ValfaPrediction_1(i) = sin(ElectricalAngle)*Vd_est_1(i)+cos(ElectricalAngle)*Vq_est_1(i);
        VbetaPrediction_1(i) =-cos(ElectricalAngle)*Vd_est_1(i)+sin(ElectricalAngle)*Vq_est_1(i);     
        
        VoltageVectorAnglePrediction_1(i) = atan2(VbetaPrediction_1(i),ValfaPrediction_1(i))+4*pi;
        VoltageVectorAnglePredictionMod_1(i) = mod(VoltageVectorAnglePrediction_1(i),pi/3);
        
     
        
        %% second prediction
        
%         Vd_est_2(i) = Rs*IdMeasured+Ls*FswOptions(i)*(idref-IdMeasured)-PolePairs*ShaftAngularSpeed*Ls*IqMeasured;
%         Vq_est_2(i) = Rs*IqMeasured+Ls*FswOptions(i)*(iqref-IqMeasured)+PolePairs*ShaftAngularSpeed*(Ld*IdMeasured+FluxPM);
        
        MagnitudePrediction_2(i) = sqrt(Vd_est_1(i)^2+Vq_est_1(i)^2);
        
        ValfaPrediction_2(i) = sin(ElectricalAngle)*Vd_est_1(i)+cos(ElectricalAngle)*Vq_est_1(i);
        VbetaPrediction_2(i) =-cos(ElectricalAngle)*Vd_est_1(i)+sin(ElectricalAngle)*Vq_est_1(i);      
        
        VoltageVectorAnglePrediction_2(i) = atan2(VbetaPrediction_2(i),ValfaPrediction_2(i))+4*pi;
        VoltageVectorAnglePredictionMod_2(i) = mod(VoltageVectorAnglePrediction_2(i),pi/3);   
        
        maPrediction_2(i) = MagnitudePrediction_2(i)/(Vdc/sqrt(3)); 
        
        SvpwmT1Prediction_2(i) = (1/FswOptions(i))*maPrediction_2(i)*sin(pi/3-VoltageVectorAnglePredictionMod_2(i));
        SvpwmT2Prediction_2(i) = (1/FswOptions(i))*maPrediction_2(i)*sin(VoltageVectorAnglePredictionMod_2(i));
        SvpwmT0Prediction_2(i) = (1/FswOptions(i))-SvpwmT1Prediction_2(i)-SvpwmT2Prediction_2(i); 
        
        VoltageDuring_T1_2(i) = 2/3*Vdc-MagnitudePrediction_2(i);
        VoltageDuring_T2_2(i) = 2/3*Vdc-MagnitudePrediction_2(i);
        VoltageDuring_T0_2(i) = -MagnitudePrediction_2(i);
        
        IqDelta_Prediction_During_T1_2(i) = -VoltageDuring_T1_2(i)*SvpwmT1Prediction_2(i)/Ls;
        IqDelta_Prediction_During_T2_2(i) = -VoltageDuring_T2_2(i)*SvpwmT2Prediction_2(i)/Ls;
        IqDelta_Prediction_During_T0_2(i) = VoltageDuring_T0_2(i)*SvpwmT0Prediction_2(i)/Ls;        
        
        IqRipplePredictionArray_2(i) = IqDelta_Prediction_During_T1_2(i)+IqDelta_Prediction_During_T2_2(i)+IqDelta_Prediction_During_T0_2(i);
        
        IdPrediction_2 = IdPrediction_1 + (1/FswOptions(i))*(Vd_est_1(i)/Ld-Rs/Ld*IdPrediction_1+Lq/Ld*PolePairs*ShaftAngularSpeed*IqPrediction_1);
        IqPrediction_2 = IqPrediction_1 + (1/FswOptions(i))*(Vq_est_1(i)/Lq-Rs/Lq*IqPrediction_1-Ld/Lq*PolePairs*ShaftAngularSpeed*IdPrediction_1-FluxPM*PolePairs*ShaftAngularSpeed/Lq);                
        
        IdPrediction_2_array(i) = IdPrediction_2;
        IqPrediction_2_array(i) = IqPrediction_2;
        
        %% calculate the cost
%         if(abs(IqPrediction_1)>30)||(abs(TePrediction_1)>50)
%             ProtectionConstant = inf;
%         else
            ProtectionConstant = 0;
%         end
%         cost(i) = (IqRipplePredictionArray_1(i)/Iq_Rated)^2*IqRippleCoeff+IqRefCoeff*((iqref-IqPrediction_1)/Iq_Rated)^2+((idref-IdPrediction_1)/Iq_Rated)^2*IdRefCoeff+ProtectionConstant+FswOptions(i)/FswMax*FswCoeff;%+IqRipplePrediction_prev^2*100000000;
        cost(i) = (IqRipplePredictionArray_2(i)/Iq_Rated)^2*IqRippleCoeff+IqRefCoeff*((iqref-IqPrediction_2)/Iq_Rated)^2+((idref-IdPrediction_2)/Iq_Rated)^2*IdRefCoeff+ProtectionConstant+FswOptions(i)/FswMax*FswCoeff;%+IqRipplePrediction_prev^2*100000000;
        if(cost(i)<MinimumCostValue)
            MinimumCostValue = cost(i);
            MinimumCostIndex = i;
        end
        
    end
    
%     [CostMinVal, MinimumCostIndex] = min(cost);
    
    DutyA = 0;
    DutyB = 0;
    DutyC = 0;
    VdsOptimum_1 = VdPrediction_2(MinimumCostIndex);
    VqsOptimum_1 = VqPrediction_2(MinimumCostIndex);
    FswSelected = FswOptions(MinimumCostIndex);
    
    Iq_1_Method1 = IqPrediction_1_array(MinimumCostIndex);
    Id_1_Method1 = IdPrediction_1_array(MinimumCostIndex);

    Iq_2_Method1 = IqPrediction_2_array(MinimumCostIndex);
    Id_2_Method1 = IdPrediction_2_array(MinimumCostIndex);
    
    VoltageVectorAngleOptimum = VoltageVectorAnglePrediction_2(MinimumCostIndex);
    TswSelected = 1/FswSelected;
    
    Vds_Optimum = Vd_est_1(MinimumCostIndex);
    Vqs_Optimum = Vq_est_1(MinimumCostIndex);

    
    Svpwm_T1 = SvpwmT1Prediction_2(MinimumCostIndex);
    Svpwm_T2 = SvpwmT2Prediction_2(MinimumCostIndex);
    Svpwm_T0 = SvpwmT0Prediction_2(MinimumCostIndex);
    
    IqRipplePrediction = IqRipplePredictionArray_2(MinimumCostIndex);
    
    if (mod(VoltageVectorAngleOptimum, 2*pi)<=pi/3)&&(mod(VoltageVectorAngleOptimum, 2*pi)>=0)  % sector 1
        DutyA = (Svpwm_T1+Svpwm_T2+Svpwm_T0/2)/TswSelected;
        DutyB = (Svpwm_T2+Svpwm_T0/2)/TswSelected;
        DutyC = (Svpwm_T0/2)/TswSelected;
%         sectornumber = 1;
        return;
    end
    if (mod(VoltageVectorAngleOptimum, 2*pi)<=2*pi/3)&&(mod(VoltageVectorAngleOptimum, 2*pi)>=pi/3)  % sector 2
        DutyA = (Svpwm_T1+Svpwm_T0/2)/TswSelected;
        DutyB = (Svpwm_T1+Svpwm_T2+Svpwm_T0/2)/TswSelected;
        DutyC = (Svpwm_T0/2)/TswSelected;
%         sectornumber = 2;
        return;
    end
    if (mod(VoltageVectorAngleOptimum, 2*pi)<=pi)&&(mod(VoltageVectorAngleOptimum, 2*pi)>=2*pi/3)  % sector 3
        if(mod(VoltageVectorAngleOptimum, pi)==0)
            DutyA = (Svpwm_T0/2)/TswSelected;
            DutyB = (Svpwm_T1+Svpwm_T0/2)/TswSelected;
            DutyC = (Svpwm_T1+Svpwm_T2+Svpwm_T0/2)/TswSelected;
        else
            DutyA = (Svpwm_T0/2)/TswSelected;
            DutyB = (Svpwm_T1+Svpwm_T2+Svpwm_T0/2)/TswSelected;
            DutyC = (Svpwm_T2+Svpwm_T0/2)/TswSelected;
        end
%         sectornumber = 3;
        return;
    end
    if (mod(VoltageVectorAngleOptimum, 2*pi)<=4*pi/3)&&(mod(VoltageVectorAngleOptimum, 2*pi)>=pi)  % sector 4
        DutyA = (Svpwm_T0/2)/TswSelected;
        DutyB = (Svpwm_T1+Svpwm_T0/2)/TswSelected;
        DutyC = (Svpwm_T1+Svpwm_T2+Svpwm_T0/2)/TswSelected;
%         sectornumber = 4;
        return;
    end
    if (mod(VoltageVectorAngleOptimum, 2*pi)<=5*pi/3)&&(mod(VoltageVectorAngleOptimum, 2*pi)>=4*pi/3)  % sector 5
        DutyA = (Svpwm_T2+Svpwm_T0/2)/TswSelected;
        DutyB = (Svpwm_T0/2)/TswSelected;
        DutyC = (Svpwm_T1+Svpwm_T2+Svpwm_T0/2)/TswSelected;
%         sectornumber = 5;
        return;
    end
    if (mod(VoltageVectorAngleOptimum, 2*pi)<=2*pi)&&(mod(VoltageVectorAngleOptimum, 2*pi)>=5*pi/3)  % sector 6
        DutyA = (Svpwm_T1+Svpwm_T2+Svpwm_T0/2)/TswSelected;
        DutyB = (Svpwm_T0/2)/TswSelected;
        DutyC = (Svpwm_T1+Svpwm_T0/2)/TswSelected;
%         sectornumber = 6;
        return;
    end
    
else %switching pulse
    iqref = iqref_prev;
    Speed_Error = Speed_Error_prev;
    FswSelected = FswSelected_prev;
    DutyA = DutyA_prev;
    DutyB = DutyB_prev;
    DutyC = DutyC_prev;
    IqRipplePrediction = IqRipplePrediction_prev;
    Vds_Optimum = Vds_Optimum_prev;
    Vqs_Optimum = Vqs_Optimum_prev;
end

== matlab function mpc_model_delayed/MATLAB Function2 ==
  data: pulse input; inputwave input; outputwave output
function outputwave  = fcn(pulse, inputwave)

persistent state

if isempty(state)
state = 0;
end

if(pulse==1)
    state = state +1;
end

if(mod(state,2)==1)
    outputwave = inputwave;
    return;
end
if(mod(state,2)==0)
    outputwave = 1-inputwave;
    return;
end

outputwave = 5;

== matlab function mpc_model_delayed/abc to dq0 ==
  data: ids output; iqs output; ias input; ibs input; ics input; ref_frame_position input; i0 output
function [ids,iqs,i0 ]  = fcn(ias,ibs,ics,ref_frame_position)





ids = 2/3*(ias*sin(ref_frame_position)+ibs*sin(ref_frame_position-2*pi/3)+ics*sin(ref_frame_position+2*pi/3));
iqs =  2/3*(ias*cos(ref_frame_position)+ibs*cos(ref_frame_position-2*pi/3)+ics*cos(ref_frame_position+2*pi/3));
i0 = 2/3*1/2*(ias+ibs+ics);
% iqs = (vqs-fluxlinkage_qs_derivative-ref_frame_velocity*fluxlinkage_ds)/rs;
% ids = (vds-fluxlinkage_ds_derivative+ref_frame_velocity*fluxlinkage_qs)/rs;

== matlab function mpc_model_delayed/MATLAB Function1 ==
  data: pulse input; inputwave input; outputwave output
function outputwave  = fcn(pulse, inputwave)

persistent state

if isempty(state)
state = 0;
end

if(pulse==1)
    state = state +1;
end

if(mod(state,2)==1)
    outputwave = inputwave;
    return;
end
if(mod(state,2)==0)
    outputwave = 1-inputwave;
    return;
end

outputwave = 5;
